simulink model "TP2_simulink"  (R2024a)
settings: Solver=VariableStepAuto  StartTime=0.0  StopTime=1.4  MaxStep=0.001  RelTol=1e-3
values from neighbouring files (symbols this model uses):
  A = [-1/(4*10^-3) -0.1/(4*10^-3) 0; 0.1/(2*10^-3) -(3*10^-3)/(2*10^-3) 0; 0 1 0]    [TP1.m]    (also in TP2.m = [0 1 0 0 0 0; -Kx/m -dx/m 0 0 0 0; 0 0 0 1 0 0; 0 0 -Ky/m -d; TP3.m = [0 1 0 0 0 0; -Kx/m -dx/m 0 0 0 0; 0 0 0 1 0 0; 0 0 -Ky/m -d)
  Aob = [0 1 0 0 0 0; -Kxobs/mobs -dxobs/mobs 0 0 0 0; 0 0 0 1 0 0; 0 0 -Kyobs/mobs -dyobs/mobs 0 0; 0 0 0 0 0 1; 0 0 0 0 -Kzobs/mobs -dzobs/mobs]    [TP2.m]
  B = [1/(4*10^-3);0;0]    [TP1.m]    (also in TP2.m = [0 0 0; 1/m 0 0; 0 0 0; 0 1/m 0; 0 0 0; 0 0 1/m]; TP3.m = [0 0 0; 1/m 0 0; 0 0 0; 0 1/m 0; 0 0 0; 0 0 1/m])
  Bob = [0 0 0; 1/mobs 0 0; 0 0 0; 0 1/mobs 0; 0 0 0; 0 0 1/mobs]    [TP2.m]
  C = [0 0 1]    [TP1.m]    (also in TP2.m = [1 0 0 0 0 0; 0 0 1 0 0 0; 0 0 0 0 1 0]; TP3.m = [1 0 0 0 0 0; 0 0 1 0 0 0; 0 0 0 0 1 0])
  L = [832330; 691770; 1550]    [TP1.m]    (also in TP2.m = (place(Aob.', C.', p)).'; TP3.m = (place(A.', C.', p)).')
settings Model: Creator=pedro.campos-afonso-  LastModifiedBy=pedro.campos-afonso-

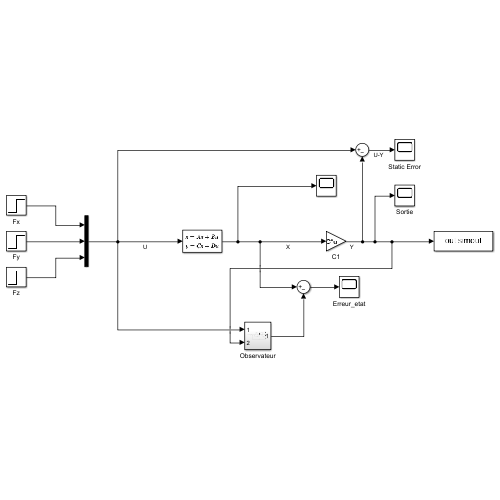
[thumbnail: Simulink's stored preview of the top-level diagram]
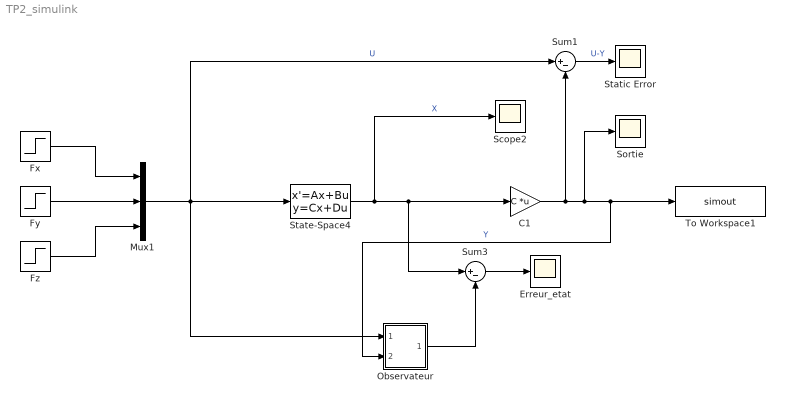
== system TP2_simulink ==
  C1 : Gain  Gain=C  Multiplication=Matrix(K*u)
  Erreur_etat : Scope
  Fx : Step  Time=0  SampleTime=0
  Fy : Step  Time=0  SampleTime=0
  Fz : Step  Time=0  SampleTime=0
  Mux1 : Mux  Inputs=3
  Observateur : Subsystem
  Scope2 : Scope
  Sortie : Scope
  State-Space4 : StateSpace  A=A  B=B  C=eye(6)  D=zeros(6,3)  InitialCondition=[0.1; 0; 0.1; 0; -0.1; 0]
  Static Error : Scope
  Sum1 : Sum  Inputs=|+-
  Sum3 : Sum  Inputs=|+-
  To Workspace1 : ToWorkspace  VariableName=simout  SaveFormat=Timeseries  SampleTime=-1
  wires:
  Fx/1 -> Mux1/1
  Fy/1 -> Mux1/2
  Fz/1 -> Mux1/3
  Mux1/1 -> Sum1/1, Observateur/1(In1), State-Space4/1  "U"
  State-Space4/1 -> Sum3/1, C1/1, Scope2/1  "X"
  C1/1 -> Sum1/2, Sortie/1, Observateur/2(In2), To Workspace1/1  "Y"
  Sum3/1 -> Erreur_etat/1
  Observateur/1(Out1) -> Sum3/2
  Sum1/1 -> Static Error/1  "U-Y"

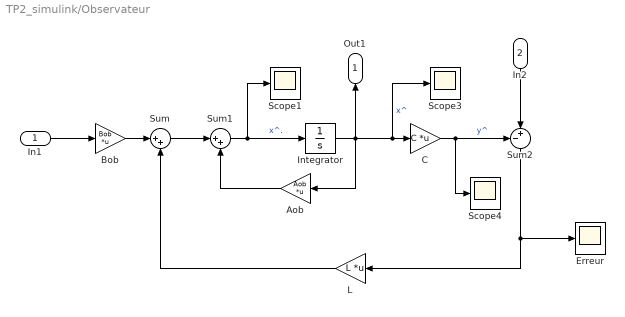
== system TP2_simulink/Observateur ==
  In1 : Inport
  In2 : Inport  Port=2
  Aob : Gain  Gain=Aob  Multiplication=Matrix(K*u) (u vector)
  Bob : Gain  Gain=Bob  Multiplication=Matrix(K*u) (u vector)
  C : Gain  Gain=C  Multiplication=Matrix(K*u) (u vector)
  Erreur : Scope
  Integrator : Integrator
  L : Gain  Gain=L  Multiplication=Matrix(K*u) (u vector)
  Scope1 : Scope
  Scope3 : Scope
  Scope4 : Scope
  Sum : Sum  Inputs=|++
  Sum1 : Sum  Inputs=|++
  Sum2 : Sum  Inputs=-+|
  Out1 : Outport
  wires:
  L/1 -> Sum/2
  Integrator/1 -> Out1/1, Aob/1, Scope3/1, C/1  "x^"
  Bob/1 -> Sum/1
  In2/1 -> Sum2/2
  Sum2/1 -> Erreur/1, L/1
  Sum/1 -> Sum1/1
  Aob/1 -> Sum1/2
  C/1 -> Sum2/1, Scope4/1  "y^"
  Sum1/1 -> Scope1/1, Integrator/1  "x^."
  In1/1 -> Bob/1
